simulink library "xrbsDSP_r4"  (Simulink 7.1)
undefined symbols (not defined in the file or in its folder): mem
libraries: xbsIndex_r4 x330
(part 2 of 5)

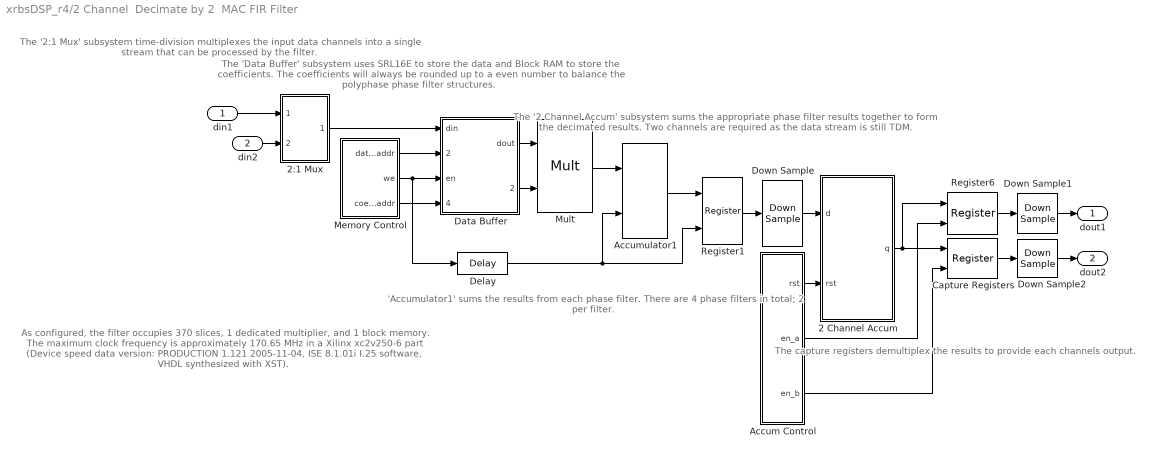
== system xrbsDSP_r4/2 Channel  Decimate by 2  MAC FIR Filter ==
  note: As configured, the  filter occupies 370 slices, 1 dedicated multiplier, and
      | 1 block memory.  The maximum clock frequency is approximately
      | 170.65 MHz in a Xilinx xc2v250-6 part (Device speed data version:
      | PRODUCTION 1.121 2005-11-04, ISE 8.1.01i I.25 software, VHDL
      | synthesized with XST).
  note: The capture registers demultiplex
      | the results to provide each
      | channels output.
  note: The '2 Channel Accum' subsystem sums the
      | appropriate phase filter results together to
      | form the decimated results.  Two channels
      | are required as the data stream is still TDM.
  note: 'Accumulator1' sums the results
      | from each phase filter.  There
      | are 4 phase filters in total; 2 per
      | filter.
  note: The 'Data Buffer' subsystem uses SRL16E to store
      | the data and Block RAM to store the
      | coefficients. The coefficients will always
      | be rounded up to a even number to balance the
      | polyphase phase filter structures.
  note: The '2:1 Mux' subsystem time-division
      | multiplexes the input data channels
      | into a single stream that can be
      | processed by the filter.
  din1 : Inport  OutDataType=sfix(16)  OutScaling=2^0
  din2 : Inport  Port=2  OutDataType=sfix(16)  OutScaling=2^0
  2 Channel Accum : Subsystem
  2:1 Mux : Subsystem
  Accum Control : Subsystem
  Accumulator1 : xbsIndex_r4/Accumulator  operation=Add  n_bits=accum2_bit_width  overflow=Wrap  scale=1  rst=on  hasbypass=on  en=off  dbl_ovrd=off  block_type=accum
      settings: infoedit="Adder or subtractor-based accumulator.   Output type and binary point position match the input.<P><P>Hardware notes: When \"Reinitialize with Input 'b' on Reset\" is selected, the accumulator is forced to run at the system rate even if the input 'b' is running at a slower rate."  xl_area=[0, 0, 0, 0, 0, 0, 0]  block_version=VER_STRING_GOES_HERE
  Capture Registers : xbsIndex_r4/Register  init=0  rst=off  en=on  dbl_ovrd=off  block_type=register
      settings: xl_area=[0, 0, 0, 0, 0, 0, 0]  block_version=VER_STRING_GOES_HERE
  Data Buffer : Subsystem
  Delay : xbsIndex_r4/Delay  en=off  latency=4  dbl_ovrd=off  reg_retiming=off  block_type=delay
      settings: infoedit="Delay line having  configurable length.<P><P>Hardware notes: A delay line is a chain, each link of which is an SRL16 followed by a flip-flop. If register retiming is enabled, the delay line is a chain of flip-flops."  xl_area=[0, 0, 0, 0, 0, 0, 0]  block_version=VER_STRING_GOES_HERE
  Down Sample : xbsIndex_r4/Down Sample  sample_ratio=length(coef)/4  sample_phase="Last Value of Frame  (most efficient)"  en=off  latency=1  dbl_ovrd=off  block_type=dsamp
      settings: xl_area=[0, 0, 0, 0, 0, 0, 0]  block_version=VER_STRING_GOES_HERE
  Down Sample1 : xbsIndex_r4/Down Sample  sample_ratio=4  sample_phase="Last Value of Frame  (most efficient)"  en=off  latency=1  dbl_ovrd=off  block_type=dsamp
      settings: xl_area=[19 37 0 0 0 0 0]  block_version=VER_STRING_GOES_HERE
  Down Sample2 : xbsIndex_r4/Down Sample  sample_ratio=4  sample_phase="Last Value of Frame  (most efficient)"  en=off  latency=1  dbl_ovrd=off  block_type=dsamp
      settings: xl_area=[19 37 0 0 0 0 0]  block_version=VER_STRING_GOES_HERE
  Memory Control : Subsystem
  Mult : xbsIndex_r4/Mult  precision=Full  arith_type="Signed  (2's comp)"  n_bits=8  bin_pt=2  quantization=Truncate  overflow=Wrap  en=off  latency=2  dbl_ovrd=off  use_behavioral_HDL=off  use_embedded=on  pipeline=on  use_rpm=off  placement_style=Rectangular shape  block_type=mult
      settings: infoedit=Multiplies two values.<P><P>Hardware notes: To use the internal pipeline stage of the dedicated multiplier you must select 'Pipeline to Greatest Extent Possible'.  xl_area=[0, 0, 0, 0, 0, 0, 0]  block_version=VER_STRING_GOES_HERE
  Register1 : xbsIndex_r4/Register  init=0  rst=off  en=on  dbl_ovrd=off  block_type=register
      settings: xl_area=[0, 0, 0, 0, 0, 0, 0]  block_version=VER_STRING_GOES_HERE
  Register6 : xbsIndex_r4/Register  init=0  rst=off  en=on  dbl_ovrd=off  block_type=register
      settings: xl_area=[0, 0, 0, 0, 0, 0, 0]  block_version=VER_STRING_GOES_HERE
  dout1 : Outport  OutDataType=sfix(16)  OutScaling=2^0
  dout2 : Outport  Port=2  OutDataType=sfix(16)  OutScaling=2^0
  wires:
  Down Sample2/1 -> dout2/1
  Down Sample1/1 -> dout1/1
  Down Sample/1 -> 2 Channel Accum/1(d)
  din2/1 -> 2:1 Mux/2(din2)
  Accum Control/3(en_b) -> Capture Registers/2
  Accum Control/2(en_a) -> Register6/2
  Accum Control/1(rst) -> 2 Channel Accum/2(rst)
  Capture Registers/1 -> Down Sample2/1
  2 Channel Accum/1(q) -> Register6/1, Capture Registers/1
  Register6/1 -> Down Sample1/1
  Accumulator1/1 -> Register1/1
  Memory Control/3(coef_addr) -> Data Buffer/4(coef_addr)
  Memory Control/2(we) -> Delay/1, Data Buffer/3(en)
  Memory Control/1(data_addr) -> Data Buffer/2(data_addr)
  Data Buffer/1(dout) -> Mult/1
  Mult/1 -> Accumulator1/1
  Delay/1 -> Accumulator1/2, Register1/2
  Register1/1 -> Down Sample/1
  Data Buffer/2(coef_out) -> Mult/2
  2:1 Mux/1(dout) -> Data Buffer/1(din)
  din1/1 -> 2:1 Mux/1(din1)

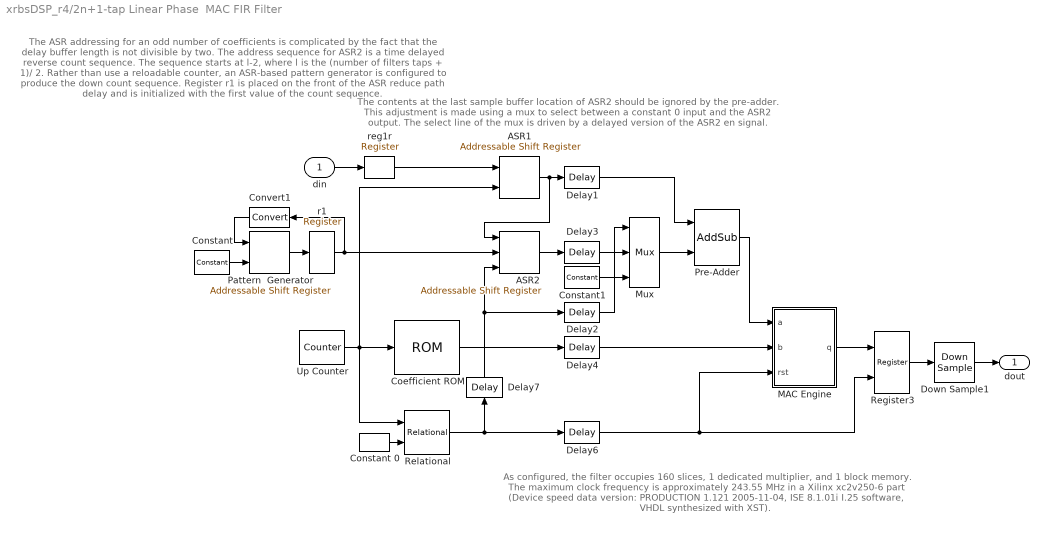
== system xrbsDSP_r4/2n+1-tap Linear Phase  MAC FIR Filter ==
  note: The ASR addressing for an odd number of coefficients is
      | complicated by the fact that the delay buffer length is not
      | divisible by two.  The address sequence for ASR2 is a time
      | delayed reverse count sequence.  The sequence starts at
      | l-2,  where l is the (number of filters taps + 1)/ 2.  Rather
      | than use a reloadable counter, an ASR-based pattern
      | generator is configured to produce the down count
      | sequence.  Register r1 is placed on the front of the ASR
      | reduce path delay and is initialized with the first value of
      | the count sequence.
  note: The contents at the last sample buffer location
      | of ASR2 should be ignored by the pre-adder.
      | This adjustment is made using a mux to select
      | between a constant 0 input and the ASR2 output.
      | The select line of the mux is driven by a delayed
      | version of the ASR2 en signal.
  note: As configured, the  filter occupies 160 slices, 1 dedicated multiplier, and
      | 1 block memory.  The maximum clock frequency is approximately
      | 243.55 MHz in a Xilinx xc2v250-6 part (Device speed data version:
      | PRODUCTION 1.121 2005-11-04, ISE 8.1.01i I.25 software, VHDL
      | synthesized with XST).
  din : Inport  OutDataType=sfix(16)  OutScaling=2^0
  ASR1 : xbsIndex_r4/Addressable Shift Register  infer_latency=on  depth=2  initVector=0  en=off  dbl_ovrd=off  use_behavioral_HDL=off  use_rpm=off  block_type=addrsr
      settings: infoedit="Delay of configurable length.  Any element in the delay line can be addressed and driven onto the output port.<P><P>Hardware notes: Implemented using SRL16s.  If a Virtex-II device is used, multiple SRLC16s are cascaded together."  xl_area=[0, 0, 0, 0, 0, 0, 0]  block_version=VER_STRING_GOES_HERE
  ASR2 : xbsIndex_r4/Addressable Shift Register  infer_latency=on  depth=2  initVector=0  en=on  dbl_ovrd=off  use_behavioral_HDL=off  use_rpm=off  block_type=addrsr
      settings: infoedit="Delay of configurable length.  Any element in the delay line can be addressed and driven onto the output port.<P><P>Hardware notes: Implemented using SRL16s.  If a Virtex-II device is used, multiple SRLC16s are cascaded together."  xl_area=[0, 0, 0, 0, 0, 0, 0]  block_version=VER_STRING_GOES_HERE
  Coefficient ROM : xbsIndex_r4/ROM  depth=(length(coef)+1)/2  initVector=coef(1:((length(coef)+1)/2))  distributed_mem=Block RAM  rst=off  init_reg=0  en=off  latency=1  arith_type="Signed  (2's comp)"  n_bits=coef_n_bits  bin_pt=coef_bin_pt  dbl_ovrd=off  use_rpm=off  block_type=sprom
      settings: xl_area=[0, 0, 0, 0, 0, 0, 0]  block_version=VER_STRING_GOES_HERE
  Constant : xbsIndex_r4/Constant  arith_type=Unsigned  const=(length(coef)+1)/2-2  n_bits=ceil(log2(((length(coef)+1)/2-1)))  bin_pt=0  explicit_period=on  period=smpl_period/((length(coef)+1)/2)  equ=P=C  opselect=C  inp2=PCIN>>17  opr=+  inp1=P  carry=CIN  dbl_ovrd=off  block_type=constant
      settings: block_version=VER_STRING_GOES_HERE
  Constant 0 : xbsIndex_r4/Constant  arith_type=Unsigned  const=0  n_bits=1  bin_pt=0  explicit_period=off  period=1  equ=P=C  opselect=C  inp2=PCIN>>17  opr=+  inp1=P  carry=CIN  dbl_ovrd=off  block_type=constant
      settings: block_version=VER_STRING_GOES_HERE
  Constant1 : xbsIndex_r4/Constant  arith_type=Unsigned  const=0  n_bits=1  bin_pt=0  explicit_period=off  period=1  equ=P=C  opselect=C  inp2=PCIN>>17  opr=+  inp1=P  carry=CIN  dbl_ovrd=off  block_type=constant
      settings: block_version=VER_STRING_GOES_HERE
  Convert1 : xbsIndex_r4/Convert  Orientation=left  arith_type=Unsigned  n_bits=ceil(log2((length(coef)+1)/2))  bin_pt=0  quantization=Truncate  overflow=Wrap  latency=0  dbl_ovrd=off  pipeline=off  block_type=convert
      settings: infoedit=The input is presented at the output after quantization and overflow effects.<P><P>Hardware notes: Additional hardware is used when rounding or saturation is selected and output width is less than the input width.  xl_area=[0, 0, 0, 0, 0, 0, 0]  block_version=VER_STRING_GOES_HERE
  Delay1 : xbsIndex_r4/Delay  en=off  latency=2  dbl_ovrd=off  reg_retiming=off  block_type=delay
      settings: infoedit="Delay line having  configurable length.<P><P>Hardware notes: A delay line is a chain, each link of which is an SRL16 followed by a flip-flop. If register retiming is enabled, the delay line is a chain of flip-flops."  xl_area=[0, 0, 0, 0, 0, 0, 0]  block_version=VER_STRING_GOES_HERE
  Delay2 : xbsIndex_r4/Delay  en=off  latency=1  dbl_ovrd=off  reg_retiming=off  block_type=delay
      settings: infoedit="Delay line having  configurable length.<P><P>Hardware notes: A delay line is a chain, each link of which is an SRL16 followed by a flip-flop. If register retiming is enabled, the delay line is a chain of flip-flops."  xl_area=[0, 0, 0, 0, 0, 0, 0]  block_version=VER_STRING_GOES_HERE
  Delay3 : xbsIndex_r4/Delay  en=off  latency=1  dbl_ovrd=off  reg_retiming=off  block_type=delay
      settings: infoedit="Delay line having  configurable length.<P><P>Hardware notes: A delay line is a chain, each link of which is an SRL16 followed by a flip-flop. If register retiming is enabled, the delay line is a chain of flip-flops."  xl_area=[0, 0, 0, 0, 0, 0, 0]  block_version=VER_STRING_GOES_HERE
  Delay4 : xbsIndex_r4/Delay  en=off  latency=2  dbl_ovrd=off  reg_retiming=off  block_type=delay
      settings: infoedit="Delay line having  configurable length.<P><P>Hardware notes: A delay line is a chain, each link of which is an SRL16 followed by a flip-flop. If register retiming is enabled, the delay line is a chain of flip-flops."  xl_area=[0, 0, 0, 0, 0, 0, 0]  block_version=VER_STRING_GOES_HERE
  Delay6 : xbsIndex_r4/Delay  en=off  latency=4  dbl_ovrd=off  reg_retiming=off  block_type=delay
      settings: infoedit="Delay line having  configurable length.<P><P>Hardware notes: A delay line is a chain, each link of which is an SRL16 followed by a flip-flop. If register retiming is enabled, the delay line is a chain of flip-flops."  xl_area=[0, 0, 0, 0, 0, 0, 0]  block_version=VER_STRING_GOES_HERE
  Delay7 : xbsIndex_r4/Delay  Orientation=up  en=off  latency=((length(coef)+1)/2)-2  dbl_ovrd=off  reg_retiming=off  block_type=delay
      settings: infoedit="Delay line having  configurable length.<P><P>Hardware notes: A delay line is a chain, each link of which is an SRL16 followed by a flip-flop. If register retiming is enabled, the delay line is a chain of flip-flops."  xl_area=[0, 0, 0, 0, 0, 0, 0]  block_version=VER_STRING_GOES_HERE
  Down Sample1 : xbsIndex_r4/Down Sample  sample_ratio=(length(coef)+1)/2  sample_phase="Last Value of Frame  (most efficient)"  en=off  latency=1  dbl_ovrd=off  block_type=dsamp
      settings: xl_area=[0, 0, 0, 0, 0, 0, 0]  block_version=VER_STRING_GOES_HERE
  MAC Engine : Subsystem
  Mux : xbsIndex_r4/Mux  inputs=2  en=off  latency=1  precision=Full  arith_type="Signed  (2's comp)"  n_bits=8  bin_pt=2  quantization=Truncate  overflow=Wrap  dbl_ovrd=off  block_type=mux
      settings: xl_area=[0, 0, 0, 0, 0, 0, 0]  block_version=VER_STRING_GOES_HERE
  Pattern  Generator : xbsIndex_r4/Addressable Shift Register  infer_latency=on  depth=2  initVector=[((length(coef)+1)/2)-1 (0:(length(coef)+1)/2-3)]  en=off  dbl_ovrd=off  use_behavioral_HDL=off  use_rpm=off  block_type=addrsr
      settings: infoedit="Delay of configurable length.  Any element in the delay line can be addressed and driven onto the output port.<P><P>Hardware notes: Implemented using SRL16s.  If a Virtex-II device is used, multiple SRLC16s are cascaded together."  xl_area=[0, 0, 0, 0, 0, 0, 0]  block_version=VER_STRING_GOES_HERE
  Pre-Adder : xbsIndex_r4/AddSub  mode=Addition  use_carryin=off  use_carryout=off  en=off  latency=1  precision=Full  arith_type=Unsigned  n_bits=8  bin_pt=2  quantization=Truncate  overflow=Wrap  dbl_ovrd=off  use_behavioral_HDL=on  pipelined=off  use_rpm=off  block_type=addsub
      settings: xl_area=[0, 0, 0, 0, 0, 0, 0]  block_version=VER_STRING_GOES_HERE
  Register3 : xbsIndex_r4/Register  init=0  rst=off  en=on  dbl_ovrd=off  block_type=register
      settings: xl_area=[0, 0, 0, 0, 0, 0, 0]  block_version=VER_STRING_GOES_HERE
  Relational : xbsIndex_r4/Relational  mode=a=b  en=off  latency=1  dbl_ovrd=off  block_type=relational
      settings: xl_area=[0, 0, 0, 0, 0, 0, 0]  block_version=VER_STRING_GOES_HERE
  Up Counter : xbsIndex_r4/Counter  cnt_type=Count Limited  cnt_to=((length(coef)+1)/2)-1  operation=Up  start_count=0  cnt_by_val=1  arith_type=Unsigned  n_bits=ceil(log2((length(coef)+1)/2))  bin_pt=0  load_pin=off  rst=off  en=off  dbl_ovrd=off  explicit_period=on  period=smpl_period/((length(coef)+1)/2)  block_type=counter
      settings: infoedit="Configurable up, down and up/down counter.<P><P>Hardware notes: Free running counters are the least expensive in hardware.  A count limited counter is implemented by combining a counter with a comparator."  xl_area=[0, 0, 0, 0, 0, 0, 0]  block_version=VER_STRING_GOES_HERE
  r1 : xbsIndex_r4/Register  init=((length(coef)+1)/2)-2  rst=off  en=off  dbl_ovrd=off  block_type=register
      settings: xl_area=[0, 0, 0, 0, 0, 0, 0]  block_version=VER_STRING_GOES_HERE
  reg1r : xbsIndex_r4/Register  init=0  rst=off  en=off  dbl_ovrd=off  block_type=register
      settings: xl_area=[0, 0, 0, 0, 0, 0, 0]  block_version=VER_STRING_GOES_HERE
  dout : Outport  OutDataType=sfix(16)  OutScaling=2^0
  wires:
  Coefficient ROM/1 -> Delay4/1
  Relational/1 -> Delay6/1, Delay7/1
  Constant 0/1 -> Relational/2
  Down Sample1/1 -> dout/1
  din/1 -> reg1r/1
  Up Counter/1 -> Relational/1, Coefficient ROM/1, ASR1/2
  ASR1/1 -> ASR2/1, Delay1/1
  reg1r/1 -> ASR1/1
  Delay1/1 -> Pre-Adder/1
  MAC Engine/1(q) -> Register3/1
  Register3/1 -> Down Sample1/1
  Pre-Adder/1 -> MAC Engine/1(a)
  Delay4/1 -> MAC Engine/2(b)
  Delay6/1 -> Register3/2, MAC Engine/3(rst)
  ASR2/1 -> Delay3/1
  Delay3/1 -> Mux/2
  Pattern  Generator/1 -> r1/1
  Constant/1 -> Pattern  Generator/2
  Convert1/1 -> Pattern  Generator/1
  Mux/1 -> Pre-Adder/2
  Constant1/1 -> Mux/3
  r1/1 -> ASR2/2, Convert1/1
  Delay7/1 -> Delay2/1, ASR2/3
  Delay2/1 -> Mux/1

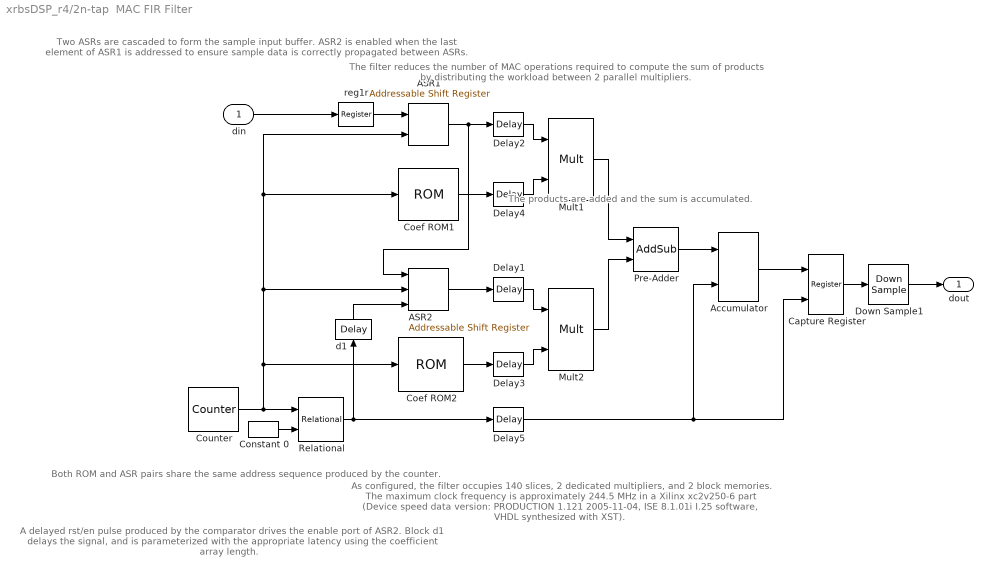
== system xrbsDSP_r4/2n-tap  MAC FIR Filter ==
  note: The filter reduces the number of MAC operations required
      | to compute the sum of products by distributing the workload
      | between 2 parallel multipliers.
  note: Both ROM and ASR pairs share the same
      | address sequence produced by the counter.
  note: The products are added and
      | the sum is accumulated.
  note: As configured, the  filter occupies 140 slices, 2 dedicated multipliers, and
      | 2 block memories.  The maximum clock frequency is approximately
      | 244.5 MHz in a Xilinx xc2v250-6 part (Device speed data version:
      | PRODUCTION 1.121 2005-11-04, ISE 8.1.01i I.25 software, VHDL
      | synthesized with XST).
  note: Two ASRs are cascaded to form the sample
      | input  buffer.  ASR2 is enabled when the last
      | element of ASR1 is addressed to ensure sample
      | data is correctly propagated between ASRs.
  note: A delayed rst/en pulse produced by the comparator
      | drives the enable port of ASR2.  Block d1 delays the
      | signal, and is parameterized with the appropriate
      | latency using the coefficient array length.
  din : Inport  OutDataType=sfix(16)  OutScaling=2^0
  ASR1 : xbsIndex_r4/Addressable Shift Register  infer_latency=on  depth=2  initVector=0  en=off  dbl_ovrd=off  use_behavioral_HDL=off  use_rpm=off  block_type=addrsr
      settings: infoedit="Delay of configurable length.  Any element in the delay line can be addressed and driven onto the output port.<P><P>Hardware notes: Implemented using SRL16s.  If a Virtex-II device is used, multiple SRLC16s are cascaded together."  xl_area=[0, 0, 0, 0, 0, 0, 0]  block_version=VER_STRING_GOES_HERE
  ASR2 : xbsIndex_r4/Addressable Shift Register  infer_latency=on  depth=2  initVector=0  en=on  dbl_ovrd=off  use_behavioral_HDL=off  use_rpm=off  block_type=addrsr
      settings: infoedit="Delay of configurable length.  Any element in the delay line can be addressed and driven onto the output port.<P><P>Hardware notes: Implemented using SRL16s.  If a Virtex-II device is used, multiple SRLC16s are cascaded together."  xl_area=[0, 0, 0, 0, 0, 0, 0]  block_version=VER_STRING_GOES_HERE
  Accumulator : xbsIndex_r4/Accumulator  operation=Add  n_bits=ceil(log2(max(1,sum(abs(coef*2^coef_bin_pt)))))+smpl_n_bits + 1  overflow=Wrap  scale=1  rst=on  hasbypass=on  en=off  dbl_ovrd=off  block_type=accum
      settings: infoedit="Adder or subtractor-based accumulator.   Output type and binary point position match the input.<P><P>Hardware notes: When \"Reinitialize with Input 'b' on Reset\" is selected, the accumulator is forced to run at the system rate even if the input 'b' is running at a slower rate."  xl_area=[0, 0, 0, 0, 0, 0, 0]  block_version=VER_STRING_GOES_HERE
  Capture Register : xbsIndex_r4/Register  init=0  rst=off  en=on  dbl_ovrd=off  block_type=register
      settings: xl_area=[0, 0, 0, 0, 0, 0, 0]  block_version=VER_STRING_GOES_HERE
  Coef ROM1 : xbsIndex_r4/ROM  depth=length(coef)/2  initVector=coef(1:(length(coef)/2))  distributed_mem=Block RAM  rst=off  init_reg=0  en=off  latency=1  arith_type="Signed  (2's comp)"  n_bits=coef_n_bits  bin_pt=coef_bin_pt  dbl_ovrd=off  use_rpm=off  block_type=sprom
      settings: xl_area=[0, 0, 0, 0, 0, 0, 0]  block_version=VER_STRING_GOES_HERE
  Coef ROM2 : xbsIndex_r4/ROM  depth=length(coef)/2  initVector=coef((length(coef)/2)+1:length(coef))  distributed_mem=Block RAM  rst=off  init_reg=0  en=off  latency=1  arith_type="Signed  (2's comp)"  n_bits=coef_n_bits  bin_pt=coef_bin_pt  dbl_ovrd=off  use_rpm=off  block_type=sprom
      settings: xl_area=[0, 0, 0, 0, 0, 0, 0]  block_version=VER_STRING_GOES_HERE
  Constant 0 : xbsIndex_r4/Constant  arith_type=Unsigned  const=0  n_bits=1  bin_pt=0  explicit_period=off  period=1  equ=P=C  opselect=C  inp2=PCIN>>17  opr=+  inp1=P  carry=CIN  dbl_ovrd=off  block_type=constant
      settings: block_version=VER_STRING_GOES_HERE
  Counter : xbsIndex_r4/Counter  cnt_type=Count Limited  cnt_to=(length(coef)/2)-1  operation=Up  start_count=0  cnt_by_val=1  arith_type=Unsigned  n_bits=ceil(log2(length(coef)/2))  bin_pt=0  load_pin=off  rst=off  en=off  dbl_ovrd=off  explicit_period=off  period=smpl_period/(length(coef)/2)  block_type=counter
      settings: infoedit="Configurable up, down and up/down counter.<P><P>Hardware notes: Free running counters are the least expensive in hardware.  A count limited counter is implemented by combining a counter with a comparator."  xl_area=[0, 0, 0, 0, 0, 0, 0]  block_version=VER_STRING_GOES_HERE
  Delay1 : xbsIndex_r4/Delay  en=off  latency=2  dbl_ovrd=off  reg_retiming=off  block_type=delay
      settings: infoedit="Delay line having  configurable length.<P><P>Hardware notes: A delay line is a chain, each link of which is an SRL16 followed by a flip-flop. If register retiming is enabled, the delay line is a chain of flip-flops."  xl_area=[0, 0, 0, 0, 0, 0, 0]  block_version=VER_STRING_GOES_HERE
  Delay2 : xbsIndex_r4/Delay  en=off  latency=2  dbl_ovrd=off  reg_retiming=off  block_type=delay
      settings: infoedit="Delay line having  configurable length.<P><P>Hardware notes: A delay line is a chain, each link of which is an SRL16 followed by a flip-flop. If register retiming is enabled, the delay line is a chain of flip-flops."  xl_area=[0, 0, 0, 0, 0, 0, 0]  block_version=VER_STRING_GOES_HERE
  Delay3 : xbsIndex_r4/Delay  en=off  latency=1  dbl_ovrd=off  reg_retiming=off  block_type=delay
      settings: infoedit="Delay line having  configurable length.<P><P>Hardware notes: A delay line is a chain, each link of which is an SRL16 followed by a flip-flop. If register retiming is enabled, the delay line is a chain of flip-flops."  xl_area=[0, 0, 0, 0, 0, 0, 0]  block_version=VER_STRING_GOES_HERE
  Delay4 : xbsIndex_r4/Delay  en=off  latency=1  dbl_ovrd=off  reg_retiming=off  block_type=delay
      settings: infoedit="Delay line having  configurable length.<P><P>Hardware notes: A delay line is a chain, each link of which is an SRL16 followed by a flip-flop. If register retiming is enabled, the delay line is a chain of flip-flops."  xl_area=[0, 0, 0, 0, 0, 0, 0]  block_version=VER_STRING_GOES_HERE
  Delay5 : xbsIndex_r4/Delay  en=off  latency=4  dbl_ovrd=off  reg_retiming=off  block_type=delay
      settings: infoedit="Delay line having  configurable length.<P><P>Hardware notes: A delay line is a chain, each link of which is an SRL16 followed by a flip-flop. If register retiming is enabled, the delay line is a chain of flip-flops."  xl_area=[0, 0, 0, 0, 0, 0, 0]  block_version=VER_STRING_GOES_HERE
  Down Sample1 : xbsIndex_r4/Down Sample  sample_ratio=length(coef)/2  sample_phase="Last Value of Frame  (most efficient)"  en=off  latency=1  dbl_ovrd=off  block_type=dsamp
      settings: xl_area=[0, 0, 0, 0, 0, 0, 0]  block_version=VER_STRING_GOES_HERE
  Mult1 : xbsIndex_r4/Mult  precision=User Defined  arith_type="Signed  (2's comp)"  n_bits=max(ceil(log2(max(1,max(abs(coef*2^coef_bin_pt)))))+smpl_n_bits + 1,smpl_bin_pt+coef_bin_pt)  bin_pt=smpl_bin_pt+coef_bin_pt  quantization=Truncate  overflow=Wrap  en=off  latency=2  dbl_ovrd=off  use_behavioral_HDL=off  use_embedded=on  pipeline=on  use_rpm=on  placement_style=Rectangular shape  block_type=mult
      settings: infoedit=Multiplies two values.<P><P>Hardware notes: To use the internal pipeline stage of the dedicated multiplier you must select 'Pipeline to Greatest Extent Possible'.  xl_area=[0, 0, 0, 0, 0, 0, 0]  block_version=VER_STRING_GOES_HERE
  Mult2 : xbsIndex_r4/Mult  precision=User Defined  arith_type="Signed  (2's comp)"  n_bits=max(ceil(log2(max(1,max(abs(coef*2^coef_bin_pt)))))+smpl_n_bits + 1,smpl_bin_pt+coef_bin_pt)  bin_pt=smpl_bin_pt+coef_bin_pt  quantization=Truncate  overflow=Wrap  en=off  latency=2  dbl_ovrd=off  use_behavioral_HDL=off  use_embedded=on  pipeline=on  use_rpm=on  placement_style=Rectangular shape  block_type=mult
      settings: infoedit=Multiplies two values.<P><P>Hardware notes: To use the internal pipeline stage of the dedicated multiplier you must select 'Pipeline to Greatest Extent Possible'.  xl_area=[0, 0, 0, 0, 0, 0, 0]  block_version=VER_STRING_GOES_HERE
  Pre-Adder : xbsIndex_r4/AddSub  mode=Addition  use_carryin=off  use_carryout=off  en=off  latency=1  precision=Full  arith_type=Unsigned  n_bits=8  bin_pt=2  quantization=Truncate  overflow=Wrap  dbl_ovrd=off  use_behavioral_HDL=on  pipelined=off  use_rpm=off  block_type=addsub
      settings: xl_area=[0, 0, 0, 0, 0, 0, 0]  block_version=VER_STRING_GOES_HERE
  Relational : xbsIndex_r4/Relational  mode=a=b  en=off  latency=1  dbl_ovrd=off  block_type=relational
      settings: xl_area=[0, 0, 0, 0, 0, 0, 0]  block_version=VER_STRING_GOES_HERE
  d1 : xbsIndex_r4/Delay  Orientation=up  en=off  latency=(length(coef)/2)-2  dbl_ovrd=off  reg_retiming=off  block_type=delay
      settings: infoedit="Delay line having  configurable length.<P><P>Hardware notes: A delay line is a chain, each link of which is an SRL16 followed by a flip-flop. If register retiming is enabled, the delay line is a chain of flip-flops."  xl_area=[0, 0, 0, 0, 0, 0, 0]  block_version=VER_STRING_GOES_HERE
  reg1r : xbsIndex_r4/Register  init=0  rst=off  en=off  dbl_ovrd=off  block_type=register
      settings: xl_area=[0, 0, 0, 0, 0, 0, 0]  block_version=VER_STRING_GOES_HERE
  dout : Outport  OutDataType=sfix(16)  OutScaling=2^0
  wires:
  Constant 0/1 -> Relational/2
  din/1 -> reg1r/1
  reg1r/1 -> ASR1/1
  Coef ROM1/1 -> Delay4/1
  ASR1/1 -> Delay2/1, ASR2/1
  ASR2/1 -> Delay1/1
  Counter/1 -> Relational/1, Coef ROM2/1, ASR2/2, ASR1/2, Coef ROM1/1
  Relational/1 -> d1/1, Delay5/1
  d1/1 -> ASR2/3
  Delay4/1 -> Mult1/2
  Delay2/1 -> Mult1/1
  Delay3/1 -> Mult2/2
  Delay1/1 -> Mult2/1
  Mult2/1 -> Pre-Adder/2
  Mult1/1 -> Pre-Adder/1
  Pre-Adder/1 -> Accumulator/1
  Delay5/1 -> Accumulator/2, Capture Register/2
  Accumulator/1 -> Capture Register/1
  Capture Register/1 -> Down Sample1/1
  Down Sample1/1 -> dout/1
  Coef ROM2/1 -> Delay3/1

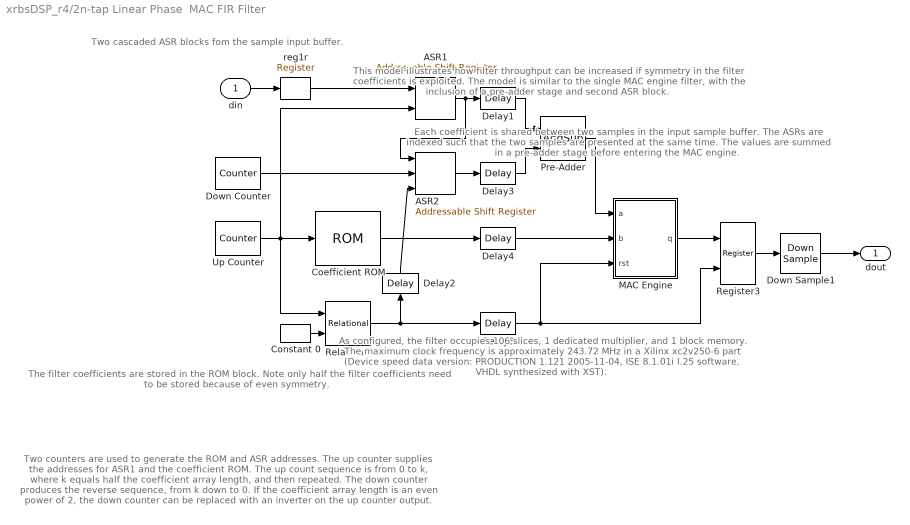
== system xrbsDSP_r4/2n-tap Linear Phase  MAC FIR Filter ==
  note: Each coefficient is shared between two samples
      | in the input sample buffer.   The ASRs are indexed
      | such that the two samples are presented at the same
      | time.  The values are summed in a pre-adder stage
      | before entering the MAC engine.
  note: Two cascaded ASR blocks fom the sample input buffer.
  note: Two counters are used to generate the ROM and ASR
      | addresses.  The up counter supplies the addresses
      | for ASR1 and the coefficient ROM.  The up count
      | sequence is from 0 to k, where k equals half the
      | coefficient array length, and then repeated.  The
      | down counter produces the reverse sequence, from
      | k down to 0.  If the coefficient array length is an even
      | power of 2, the down counter can be replaced with
      | an inverter on the up counter output.
  note: The filter coefficients are stored in the ROM block.
      | Note only half the filter coefficients need to be
      | stored because of even symmetry.
  note: As configured, the  filter occupies 106 slices, 1 dedicated multiplier, and
      | 1 block memory.  The maximum clock frequency is approximately
      | 243.72 MHz in a Xilinx xc2v250-6 part (Device speed data version: PRODUCTION 1.121 2005-11-04, ISE 8.1.01i I.25 software, VHDL synthesized with XST).
  note: This model illustrates how filter throughput can be
      | increased if symmetry in the filter coefficients is
      | exploited.  The model is similar to the single MAC
      | engine filter, with the inclusion of a pre-adder stage
      | and second ASR block.
  din : Inport  OutDataType=sfix(16)  OutScaling=2^0
  ASR1 : xbsIndex_r4/Addressable Shift Register  infer_latency=on  depth=2  initVector=0  en=off  dbl_ovrd=off  use_behavioral_HDL=off  use_rpm=off  block_type=addrsr
      settings: infoedit="Delay of configurable length.  Any element in the delay line can be addressed and driven onto the output port.<P><P>Hardware notes: Implemented using SRL16s.  If a Virtex-II device is used, multiple SRLC16s are cascaded together."  xl_area=[0, 0, 0, 0, 0, 0, 0]  block_version=VER_STRING_GOES_HERE
  ASR2 : xbsIndex_r4/Addressable Shift Register  infer_latency=on  depth=2  initVector=0  en=on  dbl_ovrd=off  use_behavioral_HDL=off  use_rpm=off  block_type=addrsr
      settings: infoedit="Delay of configurable length.  Any element in the delay line can be addressed and driven onto the output port.<P><P>Hardware notes: Implemented using SRL16s.  If a Virtex-II device is used, multiple SRLC16s are cascaded together."  xl_area=[0, 0, 0, 0, 0, 0, 0]  block_version=VER_STRING_GOES_HERE
  Coefficient ROM : xbsIndex_r4/ROM  depth=length(coef)/2  initVector=coef(1:(length(coef)/2))  rst=off  init_reg=0  en=off  latency=1  arith_type="Signed  (2's comp)"  n_bits=coef_n_bits  bin_pt=coef_bin_pt  dbl_ovrd=off  distributed_mem=Block RAM  use_rpm=off  block_type=sprom
      settings: xl_area=[0, 0, 0, 0, 0, 0, 0]  block_version=VER_STRING_GOES_HERE
  Constant 0 : xbsIndex_r4/Constant  arith_type=Unsigned  const=0  n_bits=1  bin_pt=0  explicit_period=off  period=1  equ=P=C  opselect=C  inp2=PCIN>>17  opr=+  inp1=P  carry=CIN  dbl_ovrd=off  block_type=constant
      settings: block_version=VER_STRING_GOES_HERE
  Delay1 : xbsIndex_r4/Delay  en=off  latency=1  dbl_ovrd=off  reg_retiming=off  block_type=delay
      settings: infoedit="Delay line having  configurable length.<P><P>Hardware notes: A delay line is a chain, each link of which is an SRL16 followed by a flip-flop. If register retiming is enabled, the delay line is a chain of flip-flops."  xl_area=[0, 0, 0, 0, 0, 0, 0]  block_version=VER_STRING_GOES_HERE
  Delay2 : xbsIndex_r4/Delay  Orientation=up  en=off  latency=(length(coef)/2)-2  dbl_ovrd=off  reg_retiming=off  block_type=delay
      settings: infoedit="Delay line having  configurable length.<P><P>Hardware notes: A delay line is a chain, each link of which is an SRL16 followed by a flip-flop. If register retiming is enabled, the delay line is a chain of flip-flops."  xl_area=[0, 0, 0, 0, 0, 0, 0]  block_version=VER_STRING_GOES_HERE
  Delay3 : xbsIndex_r4/Delay  en=off  latency=1  dbl_ovrd=off  reg_retiming=off  block_type=delay
      settings: infoedit="Delay line having  configurable length.<P><P>Hardware notes: A delay line is a chain, each link of which is an SRL16 followed by a flip-flop. If register retiming is enabled, the delay line is a chain of flip-flops."  xl_area=[0, 0, 0, 0, 0, 0, 0]  block_version=VER_STRING_GOES_HERE
  Delay4 : xbsIndex_r4/Delay  en=off  latency=1  dbl_ovrd=off  reg_retiming=off  block_type=delay
      settings: infoedit="Delay line having  configurable length.<P><P>Hardware notes: A delay line is a chain, each link of which is an SRL16 followed by a flip-flop. If register retiming is enabled, the delay line is a chain of flip-flops."  xl_area=[0, 0, 0, 0, 0, 0, 0]  block_version=VER_STRING_GOES_HERE
  Delay6 : xbsIndex_r4/Delay  en=off  latency=3  dbl_ovrd=off  reg_retiming=off  block_type=delay
      settings: infoedit="Delay line having  configurable length.<P><P>Hardware notes: A delay line is a chain, each link of which is an SRL16 followed by a flip-flop. If register retiming is enabled, the delay line is a chain of flip-flops."  xl_area=[0, 0, 0, 0, 0, 0, 0]  block_version=VER_STRING_GOES_HERE
  Down Counter : xbsIndex_r4/Counter  cnt_type=Count Limited  cnt_to=0  operation=Down  start_count=(length(coef)/2)-1  cnt_by_val=1  arith_type=Unsigned  n_bits=ceil(log2(length(coef)/2))  bin_pt=0  load_pin=off  rst=off  en=off  dbl_ovrd=off  explicit_period=on  period=smpl_period/(length(coef)/2)  block_type=counter
      settings: infoedit="Configurable up, down and up/down counter.<P><P>Hardware notes: Free running counters are the least expensive in hardware.  A count limited counter is implemented by combining a counter with a comparator."  xl_area=[0, 0, 0, 0, 0, 0, 0]  block_version=VER_STRING_GOES_HERE
  Down Sample1 : xbsIndex_r4/Down Sample  sample_ratio=length(coef)/2  sample_phase="Last Value of Frame  (most efficient)"  en=off  latency=1  dbl_ovrd=off  block_type=dsamp
      settings: xl_area=[0, 0, 0, 0, 0, 0, 0]  block_version=VER_STRING_GOES_HERE
  MAC Engine : Subsystem
  Pre-Adder : xbsIndex_r4/AddSub  mode=Addition  use_carryin=off  use_carryout=off  en=off  latency=1  precision=Full  arith_type=Unsigned  n_bits=8  bin_pt=2  quantization=Truncate  overflow=Wrap  dbl_ovrd=off  use_behavioral_HDL=on  pipelined=off  use_rpm=off  block_type=addsub
      settings: xl_area=[0, 0, 0, 0, 0, 0, 0]  block_version=VER_STRING_GOES_HERE
  Register3 : xbsIndex_r4/Register  init=0  rst=off  en=on  dbl_ovrd=off  block_type=register
      settings: infoedit=Delay of one sample period. <P><P>Hardware notes: Implemented using flip-flops.  xl_area=[0, 0, 0, 0, 0, 0, 0]  block_version=VER_STRING_GOES_HERE
  Relational : xbsIndex_r4/Relational  mode=a=b  en=off  latency=1  dbl_ovrd=off  block_type=relational
      settings: xl_area=[0, 0, 0, 0, 0, 0, 0]  block_version=VER_STRING_GOES_HERE
  Up Counter : xbsIndex_r4/Counter  cnt_type=Count Limited  cnt_to=(length(coef)/2)-1  operation=Up  start_count=0  cnt_by_val=1  arith_type=Unsigned  n_bits=ceil(log2(length(coef)/2))  bin_pt=0  load_pin=off  rst=off  en=off  dbl_ovrd=off  explicit_period=on  period=smpl_period/(length(coef)/2)  block_type=counter
      settings: infoedit="Configurable up, down and up/down counter.<P><P>Hardware notes: Free running counters are the least expensive in hardware.  A count limited counter is implemented by combining a counter with a comparator."  xl_area=[0, 0, 0, 0, 0, 0, 0]  block_version=VER_STRING_GOES_HERE
  reg1r : xbsIndex_r4/Register  init=0  rst=off  en=off  dbl_ovrd=off  block_type=register
      settings: infoedit=Delay of one sample period. <P><P>Hardware notes: Implemented using flip-flops.  xl_area=[0, 0, 0, 0, 0, 0, 0]  block_version=VER_STRING_GOES_HERE
  dout : Outport  OutDataType=sfix(16)  OutScaling=2^0
  wires:
  Coefficient ROM/1 -> Delay4/1
  Relational/1 -> Delay2/1, Delay6/1
  Constant 0/1 -> Relational/2
  Down Sample1/1 -> dout/1
  din/1 -> reg1r/1
  Up Counter/1 -> Relational/1, Coefficient ROM/1, ASR1/2
  ASR1/1 -> ASR2/1, Delay1/1
  reg1r/1 -> ASR1/1
  Delay1/1 -> Pre-Adder/1
  MAC Engine/1(q) -> Register3/1
  Register3/1 -> Down Sample1/1
  ASR2/1 -> Delay3/1
  Delay3/1 -> Pre-Adder/2
  Pre-Adder/1 -> MAC Engine/1(a)
  Delay2/1 -> ASR2/3
  Delay4/1 -> MAC Engine/2(b)
  Delay6/1 -> Register3/2, MAC Engine/3(rst)
  Down Counter/1 -> ASR2/2

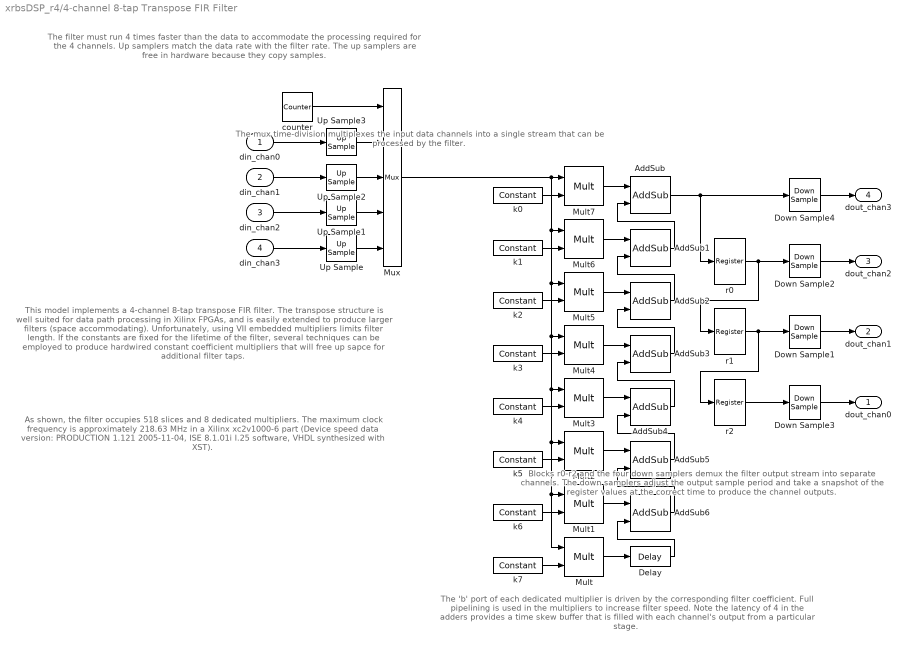
== system xrbsDSP_r4/4-channel 8-tap Transpose FIR Filter ==
  note: This model implements a 4-channel 8-tap transpose FIR filter.
      | The transpose structure is well suited for data path processing
      | in Xilinx FPGAs, and is easily extended to produce larger filters
      | (space accommodating).  Unfortunately, using VII embedded
      | multipliers limits filter length.  If the constants are fixed for the
      | lifetime of the filter, several techniques can be employed to
      | produce hardwired constant coefficient multipliers that will free
      | up sapce for additional filter taps.
  note: Blocks r0-r2 and the four down samplers
      | demux the filter output stream into separate
      | channels.  The down samplers adjust the
      | output sample period and take a snapshot
      | of the register values at the correct time to
      | produce the channel outputs.
  note: The filter must run 4 times faster than the data to
      | accommodate the processing required for the 4
      | channels.  Up samplers match the data
      | rate with the filter rate.  The up samplers are free
      | in hardware because they copy samples.
  note: The mux time-division multiplexes the input data
      | channels into a single stream that can be
      | processed by the filter.
  note: The 'b' port of each dedicated multiplier is driven by the corresponding
      | filter coefficient.  Full pipelining is used in the multipliers to increase
      | filter speed.  Note the latency of 4 in the adders provides a time skew
      | buffer that is filled with each channel's output from a particular stage.
  note: As shown, the  filter occupies 518 slices and 8 dedicated
      | multipliers. The maximum clock frequency is approximately
      | 218.63 MHz in a Xilinx xc2v1000-6 part (Device speed data
      | version: PRODUCTION 1.121 2005-11-04, ISE 8.1.01i I.25
      | software, VHDL synthesized with XST).
  din_chan0 : Inport  OutDataType=sfix(16)  OutScaling=2^0
  din_chan1 : Inport  Port=2  OutDataType=sfix(16)  OutScaling=2^0
  din_chan2 : Inport  Port=3  OutDataType=sfix(16)  OutScaling=2^0
  din_chan3 : Inport  Port=4  OutDataType=sfix(16)  OutScaling=2^0
  AddSub{,1..6} (7 alike) : xbsIndex_r4/AddSub  mode=Addition  use_carryin=off  use_carryout=off  en=off  latency=4  precision=Full  arith_type=Unsigned  n_bits=8  bin_pt=2  quantization=Truncate  overflow=Wrap  dbl_ovrd=off  use_behavioral_HDL=on  pipelined=off  use_rpm=off  block_type=addsub
      settings: xl_area=[0, 0, 0, 0, 0, 0, 0]  block_version=VER_STRING_GOES_HERE
  Delay : xbsIndex_r4/Delay  en=off  latency=4  dbl_ovrd=off  reg_retiming=off  block_type=delay
      settings: infoedit="Delay line having  configurable length.<P><P>Hardware notes: A delay line is a chain, each link of which is an SRL16 followed by a flip-flop. If register retiming is enabled, the delay line is a chain of flip-flops."  xl_area=[0, 0, 0, 0, 0, 0, 0]  block_version=VER_STRING_GOES_HERE
  Down Sample{1..4} (4 alike) : xbsIndex_r4/Down Sample  sample_ratio=4  sample_phase="Last Value of Frame  (most efficient)"  en=off  latency=1  dbl_ovrd=off  block_type=dsamp
      settings: xl_area=[0, 0, 0, 0, 0, 0, 0]  block_version=VER_STRING_GOES_HERE
  Mult{,1..7} (8 alike) : xbsIndex_r4/Mult  precision=Full  arith_type="Signed  (2's comp)"  n_bits=8  bin_pt=2  quantization=Truncate  overflow=Wrap  en=off  latency=3  dbl_ovrd=off  use_behavioral_HDL=off  use_embedded=on  pipeline=on  use_rpm=off  placement_style=Rectangular shape  block_type=mult
      settings: infoedit=Multiplies two values.<P><P>Hardware notes: To use the internal pipeline stage of the dedicated multiplier you must select 'Pipeline to Greatest Extent Possible'.  xl_area=[0, 0, 0, 0, 0, 0, 0]  block_version=VER_STRING_GOES_HERE
  Mux : xbsIndex_r4/Mux  inputs=4  en=off  latency=1  precision=Full  arith_type="Signed  (2's comp)"  n_bits=8  bin_pt=2  quantization=Truncate  overflow=Wrap  dbl_ovrd=off  block_type=mux
      settings: xl_area=[0, 0, 0, 0, 0, 0, 0]  block_version=VER_STRING_GOES_HERE
  Up Sample{,1..3} (4 alike) : xbsIndex_r4/Up Sample  sample_ratio=4  copy_samples=on  dbl_ovrd=off  block_type=usamp
      settings: infoedit="Up samples input data.  Inserted values  can be zeros or copies of the most recent input sample.<P><P>Hardware notes: No hardware is needed if inserted values are copies of the input sample; otherwise, a mux and single bit flip-flop are used."  xl_area=[0, 0, 0, 0, 0, 0, 0]  block_version=VER_STRING_GOES_HERE
  counter : xbsIndex_r4/Counter  cnt_type=Free Running  cnt_to=Inf  operation=Up  start_count=0  cnt_by_val=1  arith_type=Unsigned  n_bits=2  bin_pt=0  load_pin=off  rst=off  en=off  dbl_ovrd=off  explicit_period=off  period=smpl_period/4  block_type=counter
      settings: infoedit="Configurable up, down and up/down counter.<P><P>Hardware notes: Free running counters are the least expensive in hardware.  A count limited counter is implemented by combining a counter with a comparator."  xl_area=[0, 0, 0, 0, 0, 0, 0]  block_version=VER_STRING_GOES_HERE
  k0 : xbsIndex_r4/Constant  arith_type=Signed (2's comp)  const=coef(1)  n_bits=coef_n_bits  bin_pt=coef_bin_pt  explicit_period=off  period=1  equ=P=C  opselect=C  inp2=PCIN>>17  opr=+  inp1=P  carry=CIN  dbl_ovrd=off  block_type=constant
      settings: block_version=VER_STRING_GOES_HERE
  k1 : xbsIndex_r4/Constant  arith_type=Signed (2's comp)  const=coef(2)  n_bits=coef_n_bits  bin_pt=coef_bin_pt  explicit_period=off  period=1  equ=P=C  opselect=C  inp2=PCIN>>17  opr=+  inp1=P  carry=CIN  dbl_ovrd=off  block_type=constant
      settings: block_version=VER_STRING_GOES_HERE
  k2 : xbsIndex_r4/Constant  arith_type=Signed (2's comp)  const=coef(3)  n_bits=coef_n_bits  bin_pt=coef_bin_pt  explicit_period=off  period=1  equ=P=C  opselect=C  inp2=PCIN>>17  opr=+  inp1=P  carry=CIN  dbl_ovrd=off  block_type=constant
      settings: block_version=VER_STRING_GOES_HERE
  k3 : xbsIndex_r4/Constant  arith_type=Signed (2's comp)  const=coef(4)  n_bits=coef_n_bits  bin_pt=coef_bin_pt  explicit_period=off  period=1  equ=P=C  opselect=C  inp2=PCIN>>17  opr=+  inp1=P  carry=CIN  dbl_ovrd=off  block_type=constant
      settings: block_version=VER_STRING_GOES_HERE
  k4 : xbsIndex_r4/Constant  arith_type=Signed (2's comp)  const=coef(5)  n_bits=coef_n_bits  bin_pt=coef_bin_pt  explicit_period=off  period=1  equ=P=C  opselect=C  inp2=PCIN>>17  opr=+  inp1=P  carry=CIN  dbl_ovrd=off  block_type=constant
      settings: block_version=VER_STRING_GOES_HERE
  k5 : xbsIndex_r4/Constant  arith_type=Signed (2's comp)  const=coef(6)  n_bits=coef_n_bits  bin_pt=coef_bin_pt  explicit_period=off  period=1  equ=P=C  opselect=C  inp2=PCIN>>17  opr=+  inp1=P  carry=CIN  dbl_ovrd=off  block_type=constant
      settings: block_version=VER_STRING_GOES_HERE
  k6 : xbsIndex_r4/Constant  arith_type=Signed (2's comp)  const=coef(7)  n_bits=coef_n_bits  bin_pt=coef_bin_pt  explicit_period=off  period=1  equ=P=C  opselect=C  inp2=PCIN>>17  opr=+  inp1=P  carry=CIN  dbl_ovrd=off  block_type=constant
      settings: block_version=VER_STRING_GOES_HERE
  k7 : xbsIndex_r4/Constant  arith_type=Signed (2's comp)  const=coef(8)  n_bits=coef_n_bits  bin_pt=coef_bin_pt  explicit_period=off  period=1  equ=P=C  opselect=C  inp2=PCIN>>17  opr=+  inp1=P  carry=CIN  dbl_ovrd=off  block_type=constant
      settings: block_version=VER_STRING_GOES_HERE
  r0 : xbsIndex_r4/Register  init=0  rst=off  en=off  dbl_ovrd=off  block_type=register
      settings: xl_area=[0, 0, 0, 0, 0, 0, 0]  block_version=VER_STRING_GOES_HERE
  r1 : xbsIndex_r4/Register  init=0  rst=off  en=off  dbl_ovrd=off  block_type=register
      settings: xl_area=[0, 0, 0, 0, 0, 0, 0]  block_version=VER_STRING_GOES_HERE
  r2 : xbsIndex_r4/Register  init=0  rst=off  en=off  dbl_ovrd=off  block_type=register
      settings: xl_area=[0, 0, 0, 0, 0, 0, 0]  block_version=VER_STRING_GOES_HERE
  dout_chan0 : Outport  OutDataType=sfix(16)  OutScaling=2^0
  dout_chan1 : Outport  Port=2  OutDataType=sfix(16)  OutScaling=2^0
  dout_chan2 : Outport  Port=3  OutDataType=sfix(16)  OutScaling=2^0
  dout_chan3 : Outport  Port=4  OutDataType=sfix(16)  OutScaling=2^0
  wires:
  Mux/1 -> Mult7/1, Mult5/1, Mult4/1, Mult3/1, Mult2/1, Mult1/1, Mult/1, Mult6/1
  din_chan0/1 -> Up Sample3/1
  din_chan1/1 -> Up Sample2/1
  din_chan2/1 -> Up Sample1/1
  din_chan3/1 -> Up Sample/1
  counter/1 -> Mux/1
  Up Sample/1 -> Mux/5
  Up Sample1/1 -> Mux/4
  Up Sample2/1 -> Mux/3
  Up Sample3/1 -> Mux/2
  r0/1 -> Down Sample2/1, r1/1
  r1/1 -> Down Sample1/1, r2/1
  r2/1 -> Down Sample3/1
  Down Sample4/1 -> dout_chan3/1
  Down Sample2/1 -> dout_chan2/1
  Down Sample1/1 -> dout_chan1/1
  Down Sample3/1 -> dout_chan0/1
  AddSub/1 -> Down Sample4/1, r0/1
  Mult7/1 -> AddSub/1
  Mult6/1 -> AddSub1/1
  AddSub1/1 -> AddSub/2
  Mult5/1 -> AddSub2/1
  AddSub2/1 -> AddSub1/2
  Mult4/1 -> AddSub3/1
  AddSub3/1 -> AddSub2/2
  Mult3/1 -> AddSub4/1
  AddSub4/1 -> AddSub3/2
  Mult2/1 -> AddSub5/1
  AddSub5/1 -> AddSub4/2
  Mult1/1 -> AddSub6/1
  AddSub6/1 -> AddSub5/2
  Mult/1 -> Delay/1
  Delay/1 -> AddSub6/2
  k7/1 -> Mult/2
  k6/1 -> Mult1/2
  k5/1 -> Mult2/2
  k4/1 -> Mult3/2
  k3/1 -> Mult4/2
  k2/1 -> Mult5/2
  k1/1 -> Mult6/2
  k0/1 -> Mult7/2
